simulink model "Plant"  (R2025a)
settings: Solver=ode4  StartTime=0.0  StopTime=10  FixedStep=2e-4  RelTol=1e-3
model workspace (MAT data in the model file):
  phTyreNomPres = 262000
  plantVx0 = 68.8718280662
undefined symbols (not defined in the file): pt, sus, tyreParamVec, vp
libraries: AeroActuators x2, vehdynlibeom x1
(part 2 of 2)

== matlab function Plant/Suspension/suspStep ==
  data: Xe input; Fup output; Euler input; Ve input; pqr input; P input; Fz output; RHf output; RHr output
function [Fup, Fz, RHf, RHr] = suspStep(Xe, Euler, Ve, pqr, P)
%#codegen
% Four independent corners, SAE J670 body axes (x fwd, y RIGHT, z DOWN).
% Corner order is [FL; FR; RL; RR] -- the VDB Vehicle Body 6DOF FSusp column
% order, measured in T2.2.
%
% Rigid tyres, no unsprung mass, flat ground: a corner's suspension travel is
% just the vertical displacement of the body-fixed point above that contact
% patch. Static corner loads are carried explicitly, so compression = 0 is the
% equilibrium attitude and the model starts at rest.
%
% P = [l_f; l_r; t; hcg; kwf; kwr; cDf; cDr; kArbF; kArbR; m; g; RHf0; RHr0]

lf  = P(1);  lr  = P(2);  tw  = P(3);  hcg = P(4);
kwf = P(5);  kwr = P(6);  cDf = P(7);  cDr = P(8);
kAf = P(9);  kAr = P(10); mm  = P(11); gg  = P(12);
RHf0 = P(13); RHr0 = P(14);

phi = Euler(1); th = Euler(2);
p   = pqr(1);   q  = pqr(2);  rz = pqr(3);

% contact-patch points in body axes, relative to the CG (y RIGHT -> LEFT is -t/2)
xc = [ lf;    lf;   -lr;   -lr  ];
yc = [-tw/2;  tw/2; -tw/2;  tw/2];

sphi = sin(phi); cphi = cos(phi); sth = sin(th); cth = cos(th);

% earth-frame (z DOWN) vertical offset of each corner point from the CG, from
% the standard ZYX body->earth rotation's third row.
dz  = -sth*xc + sphi*cth*yc + cphi*cth*hcg;

% compression: POSITIVE = the body has dropped at that corner = spring compressed
del = (Xe(3) + dz) - hcg;

% exact compression rate: Euler rates from body rates (ZYX), then d(dz)/dt.
phid = p + (q*sphi + rz*cphi)*tan(th);
thd  = q*cphi - rz*sphi;
ddz  = -cth*thd*xc + (cphi*cth*phid - sphi*sth*thd)*yc ...
       + (-sphi*cth*phid - cphi*sth*thd)*hcg;
deld = Ve(3) + ddz;

% static corner loads (front axle carries l_r/l of the weight)
W   = mm*gg;
Fsf = W*lr/(2*(lf + lr));
Fsr = W*lf/(2*(lf + lr));
Fst = [Fsf; Fsf; Fsr; Fsr];
kw  = [kwf; kwf; kwr; kwr];
cD  = [cDf; cDf; cDr; cDr];

% anti-roll bars. Axle roll angle, POSITIVE = right corner compressed (right
% side down) = positive roll about +x. The bar returns a pure couple: it pushes
% the compressed corner up and pulls the extended one down, net vertical force
% zero, net roll moment -kArb*phiAxle.
phiF = (del(2) - del(1))/tw;
phiR = (del(4) - del(3))/tw;
Farb = [-kAf*phiF/tw;  kAf*phiF/tw; -kAr*phiR/tw;  kAr*phiR/tw];

% Fup = force the suspension applies to the body, POSITIVE UPWARD.
Fup = Fst + kw.*del + cD.*deld + Farb;

% tyre normal load: the same force, clamped at wheel lift (a tyre cannot pull).
Fz = max(Fup, 0);

% ride heights [mm]: vp.RHf0/vp.RHr0 are MILLIMETRES, compression is metres.
RHf = RHf0 - 1000*0.5*(del(1) + del(2));
RHr = RHr0 - 1000*0.5*(del(3) + del(4));

== matlab function Plant/Torque Path/torqueStep ==
  data: accel input; AxlTrq output; brake input; dTq input; Omega input; P input; Tbrake_applied output
function [AxlTrq, Tbrake_applied] = torqueStep(accel, brake, dTq, Omega, P)
%#codegen
% Simplified torque path. Mirrors Scripts/vehModel.m:660-663 (the pt.ATD == 0
% ladder: fixed vp.Tdist drive split, fixed vp.brkB brake split), with the
% front-axle torque-vectoring shift of simulink/ecu/tvAllocStep.m layered on.
%
% pt.ATD is NOT a Powertrain.m field -- Scripts/userOpts.m sets it -- so there is
% no ATD ladder to reproduce here; the plant is the fixed-split AWD car and the
% only per-wheel freedom is dTq (T4.2).
%
% P = [Tmax; gear; Pmax; Tdist; brkB; Tbrake_max; OmFloor]  (see the Params block
% description for the provenance of every entry).
%
% AxlTrq is [FL; FR; RL; RR] wheel-side torque [Nm], drive PLUS brake, SIGNED --
% exactly vehModel.m's T_fl..T_rr. The tyre blocks run with BrakeType = None, so
% this single signed channel is the whole wheel torque.

Tmax = P(1); gear = P(2); Pmax = P(3); Tdist = P(4);
brkB = P(5); Tbmax = P(6); OmFl = P(7);

a = min(max(accel, 0), 1);
b = min(max(brake, 0), 1);

% Lumped-machine envelope, same as Parameters/Powertrain.m:12:
%   F_tractive(v) = min(Tmax*gear/Rw, Pmax/v), here in wheel-torque terms.
% Om_motor = mean(Om_wheel)*gear (vehModel.m:655), so
%   P = T_motor*Om_motor = (T_motor*gear)*mean(Om) = T_wheel_total*mean(Om).
OmM   = max((Omega(1) + Omega(2) + Omega(3) + Omega(4))/4, OmFl);
TwCap = min(Tmax*gear, Pmax/OmM);
TwTot = a*TwCap;

% vp.Tdist is the REAR fraction (vehParams.m:20).
TwF = TwTot*(1 - Tdist);
TwR = TwTot*Tdist;

% Brake channel: identical quantity and sign to vehModel.m's T_brake decision
% variable, whose bound is [-vp.Tbrake_max, 0]. Per-wheel front torque is
% T_brake*brkB and rear is T_brake*(1-brkB), so the 4-wheel total is 2*T_brake
% and the FRONT share of it is brkB -- vehModel.m:660-663 exactly.
Tbrake_applied = -b*Tbmax;
Tbf = Tbrake_applied*brkB;
Tbr = Tbrake_applied*(1 - brkB);

% TV sign: dTq > 0 sends MORE torque to the RIGHT wheel (tvAllocStep.m:36-46).
% Corner labels are physical, so 'right' is index 2 in both frames.
AxlTrq = [TwF/2 - dTq/2 + Tbf; ...
          TwF/2 + dTq/2 + Tbf; ...
          TwR/2 + Tbr; ...
          TwR/2 + Tbr];

== matlab function Plant/Tyres PLACEHOLDER-T3.2/whlKin ==
  data: Vb input; Vxw output; pqr input; steerISO input; G input; Vyw output
function [Vxw, Vyw] = whlKin(Vb, pqr, steerISO, G)
%#codegen
% Contact-patch velocities in each WHEEL frame, [FL; FR; RL; RR].
% Body axes are SAE (y RIGHT), so v_corner = v_cg + omega x r gives
% vx - r*y and vy + r*x.
%
% STEER SIGN: DriverCmdBus.steer is ISO 8855 (+ = LEFT), the same convention and
% the same physical quantity as Scripts/vehModel.m's delta (a FRONT ROAD-WHEEL
% angle, not a hand-wheel angle). The wheel frames here are SAE, so it is
% negated exactly once, here.
%
% G = [l_f; l_r; t]

lf = G(1); lr = G(2); tw = G(3);
xc = [ lf;    lf;   -lr;   -lr  ];
yc = [-tw/2;  tw/2; -tw/2;  tw/2];

vxc = Vb(1) - pqr(3)*yc;
vyc = Vb(2) + pqr(3)*xc;

d  = -steerISO;
dl = [d; d; 0; 0];

Vxw =  vxc.*cos(dl) + vyc.*sin(dl);
Vyw = -vxc.*sin(dl) + vyc.*cos(dl);

== matlab function Plant/Tyres PLACEHOLDER-T3.2/whlFrc ==
  data: Fxw input; FxB output; Fyw input; steerISO input; FyB output
function [FxB, FyB] = whlFrc(Fxw, Fyw, steerISO)
%#codegen
% Rotate the four wheel-frame tyre forces back into SAE body axes. Inverse of
% the rotation whlKin applies to the velocities, same single negation of the
% ISO steer angle.

d  = -steerISO;
dl = [d; d; 0; 0];

FxB = Fxw.*cos(dl) - Fyw.*sin(dl);
FyB = Fxw.*sin(dl) + Fyw.*cos(dl);

== matlab function Plant/Aero/aeroStep ==
  data: Vb input; FExt output; RHf input; RHr input; aRW input; aFW input; G input; MAPF input; MAPR input; AXF input; AXR input; RWP input; FWP input; MExt output; AeroInfo output
function [FExt, MExt, AeroInfo] = aeroStep(Vb, RHf, RHr, aRW, aFW, G, ...
                                           MAPF, MAPR, AXF, AXR, RWP, FWP)
%#codegen
% LIVE RIDE-HEIGHT AERO. Codegen-safe port of simulink/aero/aeroLiveEval.m's
% formulas (T3.4). The reference file is NOT codegen-safe by design (persistent
% cache, load(), cell arrays); the arithmetic below is identical to it and is
% gate-checked against it by simulink/validation/validateAeroLive.m section (C).
%
% Ports
%   Vb    3x1  body velocity [m/s], SAE body axes (x fwd, y RIGHT, z DOWN)
%   RHf   1x1  INSTANTANEOUS front ride height [mm]  <- Suspension subsystem
%   RHr   1x1  INSTANTANEOUS rear  ride height [mm]
%   aRW   1x1  rear-wing angle  [deg] <- wing ACTUATOR POSITION (T3.4: consumed)
%   aFW   1x1  front-wing angle [deg] <- wing ACTUATOR POSITION
%   G     7x1  [rho; A; Cd0; l_f; l_r; hcg; hw]
%   MAPF  nFxnR base (Mid) FRONT lift grid, rows = RHf axis, cols = RHr axis
%   MAPR  nFxnR base (Mid) REAR  lift grid
%   AXF   nFx1 front ride-height axis [mm], ascending
%   AXR   nRx1 rear  ride-height axis [mm], ascending
%   RWP   ?xn  rear-wing blend pack  (row layout in the RWblend block description)
%   FWP   ?xn  front-wing blend pack (row layout in the FWblend block description)
%
% Outputs
%   FExt      3x1 external aero force at the CG [N], SAE axes
%   MExt      3x1 external aero moment about the CG [N.m], SAE axes
%   AeroInfo  4x1 [ClF; ClR; Cd; clampCode]
%
% SIGN CONVENTIONS (all inherited from the offline model, do not "tidy"):
%   Cl is NEGATIVE for downforce, on the fixed reference area G(2) = vp.A.
%   Body axes are SAE with z DOWN, so an axle DOWNFORCE is +z.
%   FExt acts AT THE CG, so the front/rear lift split and the wing-drag height
%   both have to be re-expressed as explicit M_y contributions. A +z force at
%   x = +l_f gives M_y = -l_f*F; a -x force at height hw above the CG gives
%   M_y = +(hw-hcg)*F. Positive M_y is NOSE UP.

rho = G(1); A = G(2); Cd0 = G(3); lf = G(4); lr = G(5); hcg = G(6); hw = G(7);

%% ---- 1) base (Mid) lift from the raw ride-height grid ------------------
% Bilinear interpolation, hand-rolled rather than interp2: identical result on
% a full rectilinear grid, codegen-safe with no toolbox dependency, and it
% gives the edge clamp (and its diagnostic flag) for free. aeroLiveEval.m and
% Functions/aeroCollapse.m:93-94 clamp to the same grid edges.
nF = numel(AXF);   nR = numel(AXR);
RHfC = min(max(RHf, AXF(1)), AXF(nF));
RHrC = min(max(RHr, AXR(1)), AXR(nR));
clampCode = 0;
if RHf < AXF(1) || RHf > AXF(nF), clampCode = clampCode + 1; end
if RHr < AXR(1) || RHr > AXR(nR), clampCode = clampCode + 2; end

iF = 1;
for k = 1:(nF-1)
    if RHfC >= AXF(k), iF = k; end
end
iR = 1;
for k = 1:(nR-1)
    if RHrC >= AXR(k), iR = k; end
end
tF = (RHfC - AXF(iF))/(AXF(iF+1) - AXF(iF));
tR = (RHrC - AXR(iR))/(AXR(iR+1) - AXR(iR));
w00 = (1-tF)*(1-tR);  w10 = tF*(1-tR);  w01 = (1-tF)*tR;  w11 = tF*tR;

ClF = w00*MAPF(iF,iR) + w10*MAPF(iF+1,iR) + w01*MAPF(iF,iR+1) + w11*MAPF(iF+1,iR+1);
ClR = w00*MAPR(iF,iR) + w10*MAPR(iF+1,iR) + w01*MAPR(iF,iR+1) + w11*MAPR(iF+1,iR+1);

%% ---- 2) rear-wing node-delta blend at aRW -----------------------------
nRW  = size(RWP,2);
aRWc = min(max(aRW, RWP(1,1)), RWP(1,nRW));
if aRW < RWP(1,1) || aRW > RWP(1,nRW), clampCode = clampCode + 4; end
LRW = cardinalWeights(RWP, aRWc);
dClF = 0; dClR = 0; dCdA = 0;
for i = 1:nRW
    dClF = dClF + LRW(i)*RWP(3,i);
    dClR = dClR + LRW(i)*RWP(4,i);
    dCdA = dCdA + LRW(i)*RWP(5,i);
end

%% ---- 3) front-wing node-delta blend at aFW ----------------------------
nFW  = size(FWP,2);
aFWc = min(max(aFW, FWP(1,1)), FWP(1,nFW));
if aFW < FWP(1,1) || aFW > FWP(1,nFW), clampCode = clampCode + 8; end
LFW = cardinalWeights(FWP, aFWc);
for i = 1:nFW
    dClF = dClF + LFW(i)*FWP(3,i);
    dClR = dClR + LFW(i)*FWP(4,i);
    dCdA = dCdA + LFW(i)*FWP(5,i);
end

ClF = ClF + dClF;
ClR = ClR + dClR;
Cd  = Cd0 + dCdA/A;

%% ---- 4) forces and moments -------------------------------------------
vx = Vb(1);
q  = 0.5*rho*A*vx*vx;
DFf = -q*ClF;                        % front axle downforce [N], + = DOWN (+z SAE)
DFr = -q*ClR;                        % rear  axle downforce [N]

% drag split, Scripts/vehModel.m:603-604: body part at hcg, wing-angle
% increment at hw. vx*abs(vx) keeps the sign right if the car ever rolls back.
vv   = vx*abs(vx);
D0   = 0.5*rho*A*Cd0*vv;             % body drag [N], + = rearward
Drw  = 0.5*rho*A*(Cd - Cd0)*vv;      % wing-increment drag [N] (may be NEGATIVE:
                                     % a low-drag wing angle has dCdA < 0)

FExt = [-(D0 + Drw); 0; DFf + DFr];
MExt = [0; -lf*DFf + lr*DFr + (hw - hcg)*Drw; 0];

AeroInfo = [ClF; ClR; Cd; clampCode];
end

% ===========================================================================
function L = cardinalWeights(P, alpha)
%#codegen
% Cardinal hermite3tanh basis weights L_i(alpha), i = 1..n. Port of
% Functions/rwBasisWeights.m's tanh switch stack (the shared owner) plus the
% Horner accumulation Functions/rwAeroMapEvalNum.m's private rwBasisNum does.
% The switches sit on the INTERIOR knots only: n-2 switches, n-1 segments.
n  = size(P,2);
wb = P(2,1);

s = zeros(1, n-2);
for k = 1:(n-2)
    s(k) = 0.5*(1 + tanh((alpha - P(1,k+1))/wb));
end

w = zeros(1, n-1);
w(1) = 1 - s(1);
acc  = s(1);
for j = 2:(n-2)
    w(j) = acc*(1 - s(j));
    acc  = acc*s(j);
end
w(n-1) = acc;

L = zeros(1, n);
for i = 1:n
    a = 0;
    for j = 1:(n-1)
        x = alpha - P(1,j);
        y = P(5 + (j-1)*4 + 1, i);
        for kk = 2:4
            y = y*x + P(5 + (j-1)*4 + kk, i);
        end
        a = a + w(j)*y;
    end
    L(i) = a;
end
end

== matlab function Plant/FSusp Assembly ==
  data: FxB input; FSusp output size=[3 4]; FyB input; Fup input
function FSusp = fsuspAssemble(FxB, FyB, Fup)
%#codegen
% VDB Vehicle Body 6DOF FSusp input: 3-by-4, rows = vehicle-fixed [x; y; z],
% columns = [FL FR RL RR]. Both MEASURED on the live R2025a block in T2.2.
%
% Row 3 is -Fup because the suspension pushes the body UP and +z is DOWN.

FSusp = [FxB(1)  FxB(2)  FxB(3)  FxB(4); ...
         FyB(1)  FyB(2)  FyB(3)  FyB(4); ...
        -Fup(1) -Fup(2) -Fup(3) -Fup(4)];
